simulink model "Scott_Connection_Y"  (R2021a)
settings: Solver=ode5  StartTime=0.0  StopTime=0.04  FixedStep=2e-6  RelTol=1e-3
InitFcn:
  | Pn1 = 5000;
  | Pn2 = 5000;
  | fg = 50;
  | V2ph_pk = 440*sqrt(2);
  | 
  | Vp1 = 440;
  | Vs1 = 220*(sqrt(3)/2);
  | rp1 = 200e-3;
  | Lp1 = 2.5e-3;
  | Rc1 = 1500;
  | Lm1 = 1500e-3;
  | 
  | Vp2 = 440;
  | Vs2 = 220*(1/2);
  | rp2 = 250e-3;
  | Lp2 = 6.5e-3;
  | Rc2 = 1200;
  | Lm2 = 1000e-3;
undefined symbols (not defined in the file): Lo_act, ro_act, Vo
libraries: dspstat3 x8, spsCurrentMeasurementLib x6, spsVoltageMeasurementLib x5, spsSeriesRLCBranchLib x3, spsLinearTransformerLib x2, spsACVoltageSourceLib x2, spspowerguiLib x1
settings Model: Creator=Triptendu  LastModifiedBy=mansi
settings SolverCC: AlgebraicLoopSolver=TrustRegion
settings DebuggingCC: SFMachineParentedDataDiag=warning

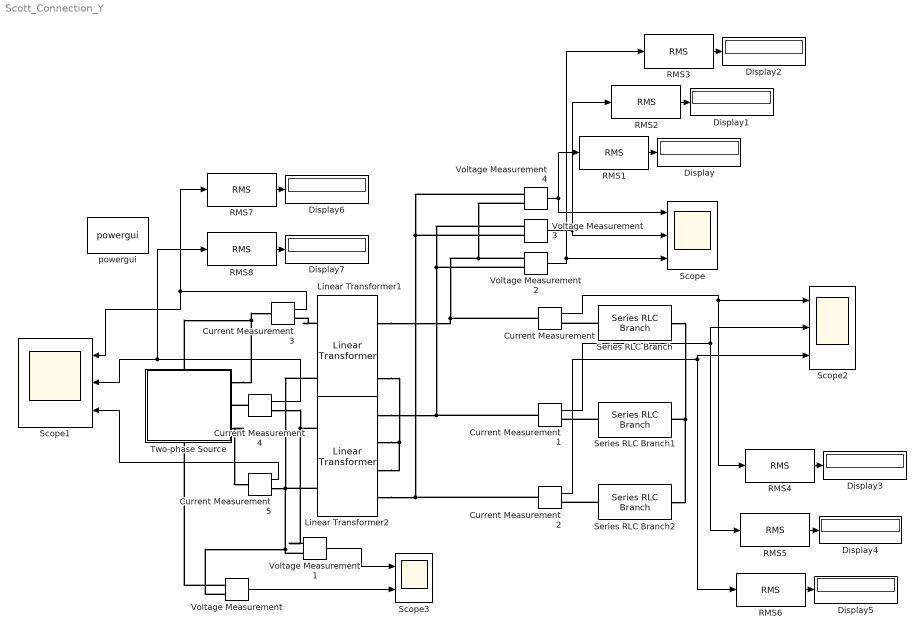
== system Scott_Connection_Y ==
  Current Measurement{,1..5} (6 alike) : spsCurrentMeasurementLib/Current Measurement  PhasorSimulation=off  OutputType=Complex  PSBequivalent=0
  Display{,1..7} (8 alike) : Display
  Linear Transformer1 : spsLinearTransformerLib/Linear Transformer  UNITS=SI  NominalPower=[5000 50]  winding1=[440 0.2 0.0025]  winding2=[381.05 1e-6 0]  ThreeWindings=off  winding3=[Vo/2 ro_act/2 Lo_act/2]  RmLm=[1500 1.5]  Measurements=None  DataType=on
  Linear Transformer2 : spsLinearTransformerLib/Linear Transformer  UNITS=SI  NominalPower=[5000 50]  winding1=[440 0.25 0.0065]  winding2=[220 1e-6 0]  ThreeWindings=on  winding3=[220 1e-6 0]  RmLm=[1200 1]  Measurements=None  DataType=on
  RMS{1..8} (8 alike) : dspstat3/RMS  run=off  directionMode=Each column  dimension=1  InputProcessing=Columns as channels (frame based)  reset_popup=None
  Scope : Scope  NumInputPorts=3
  Scope1 : Scope  NumInputPorts=3
  Scope2 : Scope  NumInputPorts=3
  Scope3 : Scope  NumInputPorts=2
  Series RLC Branch : spsSeriesRLCBranchLib/Series RLC Branch  LConnTagsString=__new0  RConnTagsString=__new0  BranchType=R  Resistance=4.84  Inductance=0  SetiL0=off  InitialCurrent=0  Capacitance=0  Setx0=off  InitialVoltage=0  Measurements=None
  Series RLC Branch1 : spsSeriesRLCBranchLib/Series RLC Branch  LConnTagsString=__new0  RConnTagsString=__new0  BranchType=R  Resistance=4.84  Inductance=0  SetiL0=off  InitialCurrent=0  Capacitance=0  Setx0=off  InitialVoltage=0  Measurements=None
  Series RLC Branch2 : spsSeriesRLCBranchLib/Series RLC Branch  LConnTagsString=__new0  RConnTagsString=__new0  BranchType=R  Resistance=4.84  Inductance=0  SetiL0=off  InitialCurrent=0  Capacitance=0  Setx0=off  InitialVoltage=0  Measurements=None
  Two-phase Source : Subsystem
  Voltage Measurement{,1..4} (5 alike) : spsVoltageMeasurementLib/Voltage Measurement  PhasorSimulation=off  OutputType=Complex  PSBequivalent=0
  powergui : spspowerguiLib/powergui  Priority=1  SimulationMode=Discrete  SampleTime=2e-6  frequency=60  Iterations=50  frequencyindice=50  Pbase=100e6  ErrMax=1e-4  UnitsV=kV  UnitsW=MW  buscounter=0  FunctionMessages=off  echomessages=off  EnableUseOfTLC=off  CurrentSourceSwitches=off  DisableSnubberDevices=off  DisableRonSwitches=off  DisableVfSwitches=off  DisplayEquations=off  AutomaticDiscreteSolvers=off  SolverType=Backward Euler  Interpol=off  ExternalGateDelay=off  methode=off  Ts=100  x0status=blocks  SPID=on  SwTol=0  HookPort=off  NonlinearTolerance=1e-4  nMaxIteration=100  ContinueOnMaxIteration=off  RestoreLinks=warning  ResistiveCurrentMeasurement=off  Frange=[0:2:500]  Ylog=off  Xlog=on  ShowGrid=off  save=off  variable=ZData  structure=0  ZoomFFT=off  StartTime=0.0  cycles=1  DisplayStyle=1  fundamental=60  FreqAxis=off  MaxFrequency=1000  frequencyindicesteady=1  RmsSteady=1  display=off
  wires:
  Current Measurement5/1 -> Scope1/3
  Voltage Measurement4/1 -> RMS1/1, Scope/1
  RMS1/1 -> Display/1
  Voltage Measurement3/1 -> RMS2/1, Scope/2
  RMS2/1 -> Display1/1
  Voltage Measurement2/1 -> RMS3/1, Scope/3
  RMS3/1 -> Display2/1
  Current Measurement/1 -> Scope2/1, RMS4/1
  RMS4/1 -> Display3/1
  Current Measurement1/1 -> Scope2/2, RMS5/1
  RMS5/1 -> Display4/1
  Current Measurement2/1 -> Scope2/3, RMS6/1
  RMS6/1 -> Display5/1
  Current Measurement3/1 -> RMS7/1, Scope1/1
  RMS7/1 -> Display6/1
  Current Measurement4/1 -> RMS8/1, Scope1/2
  RMS8/1 -> Display7/1
  Voltage Measurement1/1 -> Scope3/1
  Voltage Measurement/1 -> Scope3/2
  connections:
  Current Measurement5/RConn1 -- Linear Transformer1/LConn2 -- Linear Transformer2/LConn2 -- Voltage Measurement/LConn2 -- Voltage Measurement1/LConn2
  Linear Transformer2/RConn2 -- Linear Transformer1/RConn2 -- Linear Transformer2/RConn3
  Series RLC Branch2/RConn1 -- Series RLC Branch/RConn1 -- Series RLC Branch1/RConn1
  Current Measurement/LConn1 -- Linear Transformer1/RConn1 -- Voltage Measurement4/LConn2 -- Voltage Measurement2/LConn1
  Series RLC Branch/LConn1 -- Current Measurement/RConn1
  Current Measurement1/LConn1 -- Linear Transformer2/RConn1 -- Voltage Measurement2/LConn2 -- Voltage Measurement3/LConn1
  Series RLC Branch1/LConn1 -- Current Measurement1/RConn1
  Series RLC Branch2/LConn1 -- Current Measurement2/RConn1
  Current Measurement2/LConn1 -- Linear Transformer2/RConn4 -- Voltage Measurement3/LConn2 -- Voltage Measurement4/LConn1
  Linear Transformer1/LConn1 -- Current Measurement3/RConn1
  Current Measurement4/LConn1 -- Two-phase Source/RConn2
  Two-phase Source/RConn1 -- Current Measurement3/LConn1 -- Voltage Measurement/LConn1
  Current Measurement4/RConn1 -- Linear Transformer2/LConn1 -- Voltage Measurement1/LConn1
  Two-phase Source/RConn3 -- Current Measurement5/LConn1

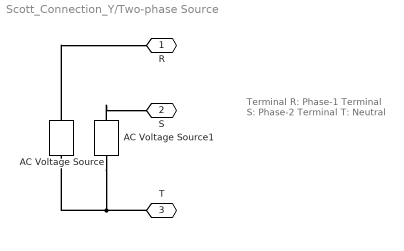
== system Scott_Connection_Y/Two-phase Source ==
  note: Terminal R: Phase-1
      | Terminal S: Phase-2
      | Terminal T: Neutral
  AC Voltage Source : spsACVoltageSourceLib/AC Voltage Source  Amplitude=440  Phase=0  Frequency=50  SampleTime=0  Measurements=None  BusType=swing  Pref=10e3  Qref=0  Qmin=-inf  Qmax=+inf
  AC Voltage Source1 : spsACVoltageSourceLib/AC Voltage Source  Amplitude=440  Phase=-90  Frequency=50  SampleTime=0  Measurements=None  BusType=swing  Pref=10e3  Qref=0  Qmin=-inf  Qmax=+inf
  R : PMIOPort  Side=Right
  S : PMIOPort  Port=2  Side=Right
  T : PMIOPort  Port=3  Side=Right
  connections:
  AC Voltage Source1/LConn1 -- T/RConn1 -- AC Voltage Source/LConn1
  AC Voltage Source1/RConn1 -- S/RConn1
  AC Voltage Source/RConn1 -- R/RConn1
